simulink library "libAircraftWeightandMassSpec"  (R2020b)
settings: Solver=VariableStepAuto  StartTime=0.0  StopTime=10.0  RelTol=1e-3
undefined symbols (not defined in the file): data
settings Model: Creator=caatay  LastModifiedBy=caatay

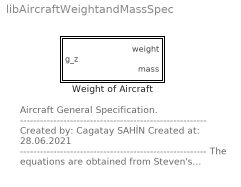
== system libAircraftWeightandMassSpec ==
  note: Aircraft General Specification.
      | --------------------------------------------------------
      | Created by: Cagatay SAHİN
      | Created at: 28.06.2021
      | --------------------------------------------------------
      | The equations are obtained from
      | Steven's textbook.
      | The reference book can be found in
      | "references folder".
      | --------------------------------------------------------
      | for question:
      | cagataysahin44@gmail.com
  Weight of Aircraft : Subsystem  mask(Aircraft Specifications - General Specifications){G=data.acSpec.general.empWeight}
      mask prompts: G "Aircraft Weight"
      mask help: Aircraft's general specifications to use in equations of motion. These specs are weight, and mass in Imperical format.
      mask Help:
      | This block is used for getting general aircraft specification such as weight and mass.
      | --------------------------------------------------------------------------------------------------------------------------------------------------
      | Input of the function:
      | 	g_z: Z-Axis gravitional acceleration (ft/s^2)
      | Output of the function:
      | 	G: Weight (lb)
      | 	m: Mass (slug)
      | --------------------------------------------------------------------------------------------------------------------------------------------------
      | All equations can be found in Steven's text book. Reference can be found in "literature" subfolder.
      | for question: "cagataysahin44@gmail.com"
      mask Display:
      | port_label('output',1,'G','texmode','on');
      | port_label('output',2,'m','texmode','on');

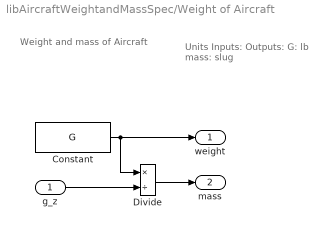
== system libAircraftWeightandMassSpec/Weight of Aircraft ==
  note: Weight and mass of Aircraft
  note: Units
      | Inputs:
      |
      | Outputs:
      | G: lb
      | mass: slug
  g_z : Inport
  Constant : Constant  Value=G
  Divide : Product  Inputs=*/
  weight : Outport  VectorParamsAs1DForOutWhenUnconnected=off
  mass : Outport  Port=2  VectorParamsAs1DForOutWhenUnconnected=off
  wires:
  Constant/1 -> Divide/1, weight/1
  g_z/1 -> Divide/2
  Divide/1 -> mass/1
